simulink model "Project2"  (R2015a)
settings: Solver=ode45  StartTime=0.0  StopTime=10000  RelTol=1e-3
PreLoadFcn:
  | Init
InitFcn:
  | Init
values from neighbouring files (symbols this model uses):
  a = 5    [Init.m]
  b = 10    [Init.m]
  PACCPrecision = 32    [Init.m]
  seed = [1,2,3,4,5,6]    [Init.m]
undefined symbols (not defined in the file or in its folder): c
libraries: xbsIndex_r4 x91, xrbsComm_r4 x1
(part 1 of 2)
settings Model: Creator=chrisd  LastModifiedBy=kchilds
settings DataIOCC: SignalLoggingSaveFormat=ModelDataLogs  SignalLoggingName=sigsOut
settings OptimizationCC: BlockReduction=off  BooleanDataType=off  ExpressionDepthLimit=2147483647  InitFltsAndDblsToZero=on
settings DebuggingCC: SaveWithParameterizedLinksMsg=none  UnderspecifiedInitializationDetection=Classic  MergeDetectMultiDrivingBlocksExec=none  SignalResolutionControl=TryResolveAllWithWarning  MultiTaskDSMMsg=warning  MultiTaskCondExecSysMsg=none  FcnCallInpInsideContextMsg=UseLocalSettings  StateNameClashWarn=warning
settings HardwareCC: TargetUnknown=on
settings GRTTargetCC: TargetFcnLib=ansi_tfl_tmw.mat  ModelReferenceCompliant=off  CombineOutputUpdateFcns=off  MatFileLogging=off  GRTInterface=on

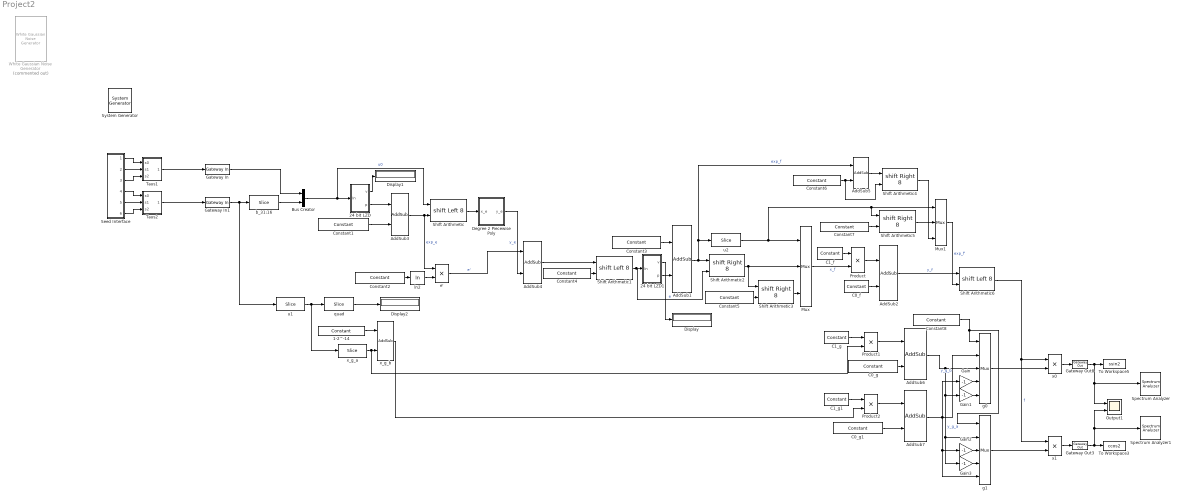
== system Project2 ==
  " System Generator" : xbsIndex_r4/ System Generator  Tag=genX  xilinxfamily=kintex7  part=xc7k325t  speed=-3  package=fbg676  synthesis_tool=Vivado  clock_wrapper=Clock Enables  directory=C:/xilinx_projects/matlab/ddc/gc4016/DDS/xilinx  proj_type=Project Navigator  Synth_file=Vivado Synthesis Defaults  Impl_file=Vivado Implementation Defaults  testbench=off  simulink_period=1  sysclk_period=7.14  dcm_input_clock_period=100  incr_netlist=off  trim_vbits=According to Block Masks  dbl_ovrd=According to Block Masks  core_generation=According to Block Masks  run_coregen=off  deprecated_control=off  eval_field=0  block_type=sysgen
      settings: block_version=12.2
  1-2^-14 : xbsIndex_r4/Constant  const=1-2^-14  gui_display_data_type=Fixed-point  arith_type=Signed (2's comp)  n_bits=LUTPrecision  bin_pt=LUTPrecisionFrc  preci_type=Single  exp_width=8  frac_width=24  explicit_period=off  period=1  equ=P=C  opselect=C  inp2=PCIN>>17  opr=+  inp1=P  carry=CIN  dbl_ovrd=off  block_type=constant
      settings: block_version=12.2
  24 bit LZD : Subsystem
  24 bit LZD1 : Subsystem
  AddSub1 : xbsIndex_r4/AddSub  mode=Subtraction  use_carryin=off  use_carryout=off  en=off  latency=0  precision=User Defined  arith_type="Signed  (2's comp)"  n_bits=nBitsIntDDSOutput  bin_pt=nBitsIntDDSOutputFrc  quantization=Truncate  overflow=Wrap  use_behavioral_HDL=off  hw_selection=Fabric  pipelined=off  dbl_ovrd=off  block_type=addsub
      settings: block_version=12.2
  AddSub{2..3,5..7} (5 alike) : xbsIndex_r4/AddSub  mode=Addition  use_carryin=off  use_carryout=off  en=off  latency=0  precision=User Defined  arith_type="Signed  (2's comp)"  n_bits=nBitsIntDDSOutput  bin_pt=nBitsIntDDSOutputFrc  quantization=Truncate  overflow=Wrap  use_behavioral_HDL=off  hw_selection=Fabric  pipelined=off  dbl_ovrd=off  block_type=addsub
      settings: block_version=12.2
  AddSub4 : xbsIndex_r4/AddSub  mode=Subtraction  use_carryin=off  use_carryout=off  en=off  latency=0  precision=User Defined  arith_type="Signed  (2's comp)"  n_bits=nBitsIntDDSOutput  bin_pt=nBitsIntDDSOutputFrc  quantization=Truncate  overflow=Wrap  use_behavioral_HDL=off  hw_selection=Fabric  pipelined=off  dbl_ovrd=off  block_type=addsub
      settings: block_version=12.2
  Bus Creator : BusCreator  Inputs=2
  C0_f : xbsIndex_r4/Constant  const=0  gui_display_data_type=Fixed-point  arith_type=Signed (2's comp)  n_bits=LUTPrecision  bin_pt=LUTPrecisionFrc  preci_type=Single  exp_width=8  frac_width=24  explicit_period=off  period=1  equ=P=C  opselect=C  inp2=PCIN>>17  opr=+  inp1=P  carry=CIN  dbl_ovrd=off  block_type=constant
      settings: block_version=12.2
  C0_g : xbsIndex_r4/Constant  const=1  gui_display_data_type=Fixed-point  arith_type=Signed (2's comp)  n_bits=LUTPrecision  bin_pt=LUTPrecisionFrc  preci_type=Single  exp_width=8  frac_width=24  explicit_period=off  period=1  equ=P=C  opselect=C  inp2=PCIN>>17  opr=+  inp1=P  carry=CIN  dbl_ovrd=off  block_type=constant
      settings: block_version=12.2
  C0_g1 : xbsIndex_r4/Constant  const=1  gui_display_data_type=Fixed-point  arith_type=Signed (2's comp)  n_bits=LUTPrecision  bin_pt=LUTPrecisionFrc  preci_type=Single  exp_width=8  frac_width=24  explicit_period=off  period=1  equ=P=C  opselect=C  inp2=PCIN>>17  opr=+  inp1=P  carry=CIN  dbl_ovrd=off  block_type=constant
      settings: block_version=12.2
  C1_f : xbsIndex_r4/Constant  const=0  gui_display_data_type=Fixed-point  arith_type=Signed (2's comp)  n_bits=LUTPrecision  bin_pt=LUTPrecisionFrc  preci_type=Single  exp_width=8  frac_width=24  explicit_period=off  period=1  equ=P=C  opselect=C  inp2=PCIN>>17  opr=+  inp1=P  carry=CIN  dbl_ovrd=off  block_type=constant
      settings: block_version=12.2
  C1_g : xbsIndex_r4/Constant  const=0  gui_display_data_type=Fixed-point  arith_type=Signed (2's comp)  n_bits=LUTPrecision  bin_pt=LUTPrecisionFrc  preci_type=Single  exp_width=8  frac_width=24  explicit_period=off  period=1  equ=P=C  opselect=C  inp2=PCIN>>17  opr=+  inp1=P  carry=CIN  dbl_ovrd=off  block_type=constant
      settings: block_version=12.2
  C1_g1 : xbsIndex_r4/Constant  const=0  gui_display_data_type=Fixed-point  arith_type=Signed (2's comp)  n_bits=LUTPrecision  bin_pt=LUTPrecisionFrc  preci_type=Single  exp_width=8  frac_width=24  explicit_period=off  period=1  equ=P=C  opselect=C  inp2=PCIN>>17  opr=+  inp1=P  carry=CIN  dbl_ovrd=off  block_type=constant
      settings: block_version=12.2
  Constant{1,4..8} (6 alike) : xbsIndex_r4/Constant  const=1  gui_display_data_type=Fixed-point  arith_type=Signed (2's comp)  n_bits=LUTPrecision  bin_pt=LUTPrecisionFrc  preci_type=Single  exp_width=8  frac_width=24  explicit_period=off  period=1  equ=P=C  opselect=C  inp2=PCIN>>17  opr=+  inp1=P  carry=CIN  dbl_ovrd=off  block_type=constant
      settings: block_version=12.2
  Constant2 : xbsIndex_r4/Constant  const=2  gui_display_data_type=Fixed-point  arith_type=Signed (2's comp)  n_bits=LUTPrecision  bin_pt=LUTPrecisionFrc  preci_type=Single  exp_width=8  frac_width=24  explicit_period=off  period=1  equ=P=C  opselect=C  inp2=PCIN>>17  opr=+  inp1=P  carry=CIN  dbl_ovrd=off  block_type=constant
      settings: block_version=12.2
  Constant3 : xbsIndex_r4/Constant  const=5  gui_display_data_type=Fixed-point  arith_type=Signed (2's comp)  n_bits=LUTPrecision  bin_pt=LUTPrecisionFrc  preci_type=Single  exp_width=8  frac_width=24  explicit_period=off  period=1  equ=P=C  opselect=C  inp2=PCIN>>17  opr=+  inp1=P  carry=CIN  dbl_ovrd=off  block_type=constant
      settings: block_version=12.2
  Degree 2 Piecewise Poly : Subsystem
  Display : Display
      settings: Format=binary (Stored Integer)
  Display1 : Display
      settings: Format=binary (Stored Integer)
  Display2 : Display
      settings: Format=binary (Stored Integer)
  Gain{,1..3} (4 alike) : Gain  Gain=-1
  Gateway In : xbsIndex_r4/Gateway In  gui_display_data_type=Fixed-point  arith_type="Signed  (2's comp)"  n_bits=32  bin_pt=0  preci_type=Single  exp_width=8  frac_width=24  rows=1  columns=1  quantization="Round  (unbiased: +/- Inf)"  overflow=Saturate  period=1  UseAsADC=off  ADCChannel='1'  interface=None  automatic_assignment=on  address_offset=hex2dec('00')  intf_name=''  intf_description=''  timing_constraint=None  locs_specified=off  LOCs={}  io_standard={}  inherit_from_input=off  hdl_port=on  dbl_ovrd=off  block_type=gatewayin
      settings: xl_area=[0, 0, 0, 0, 0, 0, 0]  block_version=VER_STRING_GOES_HERE
  Gateway In1 : xbsIndex_r4/Gateway In  gui_display_data_type=Fixed-point  arith_type="Signed  (2's comp)"  n_bits=32  bin_pt=0  preci_type=Single  exp_width=8  frac_width=24  rows=1  columns=1  quantization="Round  (unbiased: +/- Inf)"  overflow=Saturate  period=1  UseAsADC=off  ADCChannel='1'  interface=None  automatic_assignment=on  address_offset=hex2dec('00')  intf_name=''  intf_description=''  timing_constraint=None  locs_specified=off  LOCs={}  io_standard={}  inherit_from_input=off  hdl_port=on  dbl_ovrd=off  block_type=gatewayin
      settings: xl_area=[0, 0, 0, 0, 0, 0, 0]  block_version=VER_STRING_GOES_HERE
  Gateway Out3 : xbsIndex_r4/Gateway Out  inherit_from_input=off  hdl_port=on  rows=1  columns=1  UseAsDAC=off  DACChannel='1'  interface=None  automatic_assignment=on  address_offset=hex2dec('00')  intf_name=''  intf_description=''  timing_constraint=None  locs_specified=off  LOCs={}  io_standard={}  block_type=gatewayout
      settings: infoedit="Gateway out block.  Converts Xilinx fixed point inputs into ouputs of type Simulink integer, double, or fixed point.<P><P>Hardware notes:  In hardware these blocks become top level output ports or are discarded, depending on how they are configured."  xl_area=[0, 0, 0, 0, 0, 0, 0]  block_version=VER_STRING_GOES_HERE
  Gateway Out8 : xbsIndex_r4/Gateway Out  inherit_from_input=off  hdl_port=on  rows=1  columns=1  UseAsDAC=off  DACChannel='1'  interface=None  automatic_assignment=on  address_offset=hex2dec('00')  intf_name=''  intf_description=''  timing_constraint=None  locs_specified=off  LOCs={}  io_standard={}  block_type=gatewayout
      settings: infoedit="Gateway out block.  Converts Xilinx fixed point inputs into ouputs of type Simulink integer, double, or fixed point.<P><P>Hardware notes:  In hardware these blocks become top level output ports or are discarded, depending on how they are configured."  xl_area=[0, 0, 0, 0, 0, 0, 0]  block_version=VER_STRING_GOES_HERE
  Mux : xbsIndex_r4/Mux  inputs=2  en=off  latency=0  precision=Full  arith_type=Unsigned  n_bits=16  bin_pt=14  quantization=Truncate  overflow=Wrap  dbl_ovrd=off  block_type=mux
  Mux1 : xbsIndex_r4/Mux  inputs=2  en=off  latency=0  precision=Full  arith_type=Unsigned  n_bits=16  bin_pt=14  quantization=Truncate  overflow=Wrap  dbl_ovrd=off  block_type=mux
  Output1 : Scope  NumInputPorts=2
      settings: TimeRange=5000  YMin=-200000~-200000  YMax=200000~200000
  Product : Product
  Product1 : Product
  Product2 : Product
  Seed Interface : Subsystem
  Shift Arithmetic : ArithShift  BitShiftNumberSource=Input port  BitShiftNumber=8  BitShiftDirection=Left  DiagnosticForOORShift=Warning  CheckOORBitShift=on
      settings: InputPortMap=u0,p1
  Shift Arithmetic1 : ArithShift  BitShiftNumberSource=Input port  BitShiftNumber=8  BitShiftDirection=Left  DiagnosticForOORShift=Warning  CheckOORBitShift=on
      settings: InputPortMap=u0,p1
  Shift Arithmetic{2..5} (4 alike) : ArithShift  BitShiftNumberSource=Input port  BitShiftNumber=8  BitShiftDirection=Right  DiagnosticForOORShift=Warning  CheckOORBitShift=on
      settings: InputPortMap=u0,p1
  Shift Arithmetic6 : ArithShift  BitShiftNumberSource=Input port  BitShiftNumber=8  BitShiftDirection=Left  DiagnosticForOORShift=Warning  CheckOORBitShift=on
      settings: InputPortMap=u0,p1
  Spectrum Analyzer : SpectrumAnalyzer
  Spectrum Analyzer1 : SpectrumAnalyzer
  Taus1 : Subsystem
  Taus2 : Subsystem
  To Workspace3 : ToWorkspace  VariableName=ccos2  SaveFormat=Structure  SampleTime=-1
  To Workspace5 : ToWorkspace  VariableName=ssin2  SaveFormat=Structure  SampleTime=-1
  White Gaussian Noise Generator : xrbsComm_r4/White Gaussian  Noise Generator  Commented=on  seed=512
  b_31:16 : xbsIndex_r4/Slice  nbits=16  boolean_output=off  mode=Upper Bit Location + Width  bit1=0  base1=LSB of Input  bit0=PACCPrecision-1  base0=LSB of Input  dbl_ovrd=off  block_type=slice
      settings: block_version=12.2
  e' : Product
  g0 : xbsIndex_r4/Mux  inputs=4  en=off  latency=0  precision=Full  arith_type=Unsigned  n_bits=16  bin_pt=14  quantization=Truncate  overflow=Wrap  dbl_ovrd=off  block_type=mux
  g1 : xbsIndex_r4/Mux  inputs=4  en=off  latency=0  precision=Full  arith_type=Unsigned  n_bits=16  bin_pt=14  quantization=Truncate  overflow=Wrap  dbl_ovrd=off  block_type=mux
  ln2 : Math  Operator=log  OutputSignalType=real  SaturateOnIntegerOverflow=on
  quad : xbsIndex_r4/Slice  nbits=2  boolean_output=off  mode=Upper Bit Location + Width  bit1=0  base1=MSB of Input  bit0=0  base0=LSB of Input  dbl_ovrd=off  block_type=slice
      settings: block_version=12.2
  u1 : xbsIndex_r4/Slice  nbits=16  boolean_output=off  mode=Lower Bit Location + Width  bit1=0  base1=MSB of Input  bit0=0  base0=LSB of Input  dbl_ovrd=off  block_type=slice
      settings: block_version=12.2
  u2 : xbsIndex_r4/Slice  nbits=1  boolean_output=off  mode=Upper Bit Location + Width  bit1=0  base1=MSB of Input  bit0=0  base0=LSB of Input  dbl_ovrd=off  block_type=slice
      settings: block_version=12.2
  x0 : Product
  x1 : Product
  x_g_a : xbsIndex_r4/Slice  nbits=14  boolean_output=off  mode=Lower Bit Location + Width  bit1=0  base1=MSB of Input  bit0=0  base0=LSB of Input  dbl_ovrd=off  block_type=slice
      settings: block_version=12.2
  x_g_b : xbsIndex_r4/AddSub  mode=Subtraction  use_carryin=off  use_carryout=off  en=off  latency=0  precision=User Defined  arith_type="Signed  (2's comp)"  n_bits=nBitsIntDDSOutput  bin_pt=nBitsIntDDSOutputFrc  quantization=Truncate  overflow=Wrap  use_behavioral_HDL=off  hw_selection=Fabric  pipelined=off  dbl_ovrd=off  block_type=addsub
      settings: block_version=12.2
  wires:
  Gateway Out8/1 -> Spectrum Analyzer/1, Output1/1, To Workspace5/1
  Gateway In1/1 -> b_31:16/1, u1/1
  Gateway In/1 -> Bus Creator/1
  b_31:16/1 -> Bus Creator/2
  Bus Creator/1 -> Shift Arithmetic/1, 24 bit LZD/1(In)  "u0"
  Constant1/1 -> AddSub3/2
  24 bit LZD/2(p) -> AddSub3/1
  AddSub3/1 -> e'/1, Shift Arithmetic/2  "exp_e"
  Shift Arithmetic/1 -> Degree 2 Piecewise Poly/1(x_e)
  Constant2/1 -> ln2/1
  ln2/1 -> e'/2
  Degree 2 Piecewise Poly/1(y_e) -> AddSub4/2  "y_e"
  e'/1 -> AddSub4/1  "e'"
  24 bit LZD1/2(p) -> AddSub1/2
  Constant3/1 -> AddSub1/1
  AddSub4/1 -> Shift Arithmetic1/1
  Constant4/1 -> Shift Arithmetic1/2
  Shift Arithmetic1/1 -> Shift Arithmetic2/2, 24 bit LZD1/1(In)  "e"
  AddSub1/1 -> AddSub5/1, u2/1, Shift Arithmetic2/1  "exp_f"
  u2/1 -> Shift Arithmetic5/1, Mux1/1, Mux/1
  Constant5/1 -> Shift Arithmetic3/2
  Shift Arithmetic2/1 -> Mux/2, Shift Arithmetic3/1
  Shift Arithmetic3/1 -> Mux/3
  Mux/1 -> Product/2  "x_f"
  Product/1 -> AddSub2/1
  AddSub2/1 -> Shift Arithmetic6/1  "y_f"
  C0_f/1 -> AddSub2/2
  C1_f/1 -> Product/1
  Constant6/1 -> Shift Arithmetic4/2, AddSub5/2
  AddSub5/1 -> Shift Arithmetic4/1
  Shift Arithmetic4/1 -> Mux1/3
  Shift Arithmetic5/1 -> Mux1/2
  Constant7/1 -> Shift Arithmetic5/2
  Mux1/1 -> Shift Arithmetic6/2  "exp_f'"
  Shift Arithmetic6/1 -> x1/1, x0/1  "f"
  u1/1 -> x_g_a/1, quad/1
  1-2^-14/1 -> x_g_b/1
  Product1/1 -> AddSub6/1
  x_g_a/1 -> Product1/2, x_g_b/2
  C1_g/1 -> Product1/1
  C0_g/1 -> AddSub6/2
  AddSub6/1 -> Gain1/1, Gain3/1, g1/2, g0/3  "y_g_a"
  Product2/1 -> AddSub7/1
  x_g_b/1 -> Product2/2
  C1_g1/1 -> Product2/1
  C0_g1/1 -> AddSub7/2
  AddSub7/1 -> Gain/1, Gain2/1, g1/5, g0/2  "y_g_b"
  Gain/1 -> g0/4
  Gain1/1 -> g0/5
  Gain2/1 -> g1/3
  Gain3/1 -> g1/4
  g0/1 -> x0/2
  g1/1 -> x1/2
  x0/1 -> Gateway Out8/1
  x1/1 -> Gateway Out3/1
  Gateway Out3/1 -> Spectrum Analyzer1/1, Output1/2, To Workspace3/1
  24 bit LZD1/1(v) -> Display/1
  24 bit LZD/1(v) -> Display1/1
  quad/1 -> Display2/1
  Constant8/1 -> g0/1, g1/1
  Taus1/1(taus) -> Gateway In/1
  Taus2/1(taus) -> Gateway In1/1
  Seed Interface/2(Seed2) -> Taus1/2(s1)
  Seed Interface/1(Seed1) -> Taus1/1(s0)
  Seed Interface/3(Seed3) -> Taus1/3(s2)
  Seed Interface/4(Seed4) -> Taus2/1(s0)
  Seed Interface/5(Seed5) -> Taus2/2(s1)
  Seed Interface/6(Seed6) -> Taus2/3(s2)

== system Project2/24 bit LZD ==
  In : Inport
  16 bit LZD : Subsystem
  8 bit LZD : Subsystem
  Bus Creator1 : BusCreator  Inputs=2
  Demux : Demux  Outputs=24
  Logical Operator : Logic  Operator=OR  IconShape=distinctive  AllPortsSameDT=off  OutDataTypeStr=boolean
  Logical Operator2 : Logic  Operator=NOT  IconShape=distinctive  AllPortsSameDT=off  OutDataTypeStr=boolean
  Mux : Mux  Inputs=2
  v : Outport
  p : Outport  Port=2
  wires:
  Demux/8 -> 16 bit LZD/8(a7)
  Demux/10 -> 16 bit LZD/10(a9)
  In/1 -> Demux/1
  Demux/14 -> 16 bit LZD/14(a13)
  Demux/17 -> 8 bit LZD/1(a0)
  Demux/2 -> 16 bit LZD/2(a1)
  Demux/7 -> 16 bit LZD/7(a6)
  Demux/15 -> 16 bit LZD/15(a14)
  Demux/6 -> 16 bit LZD/6(a5)
  Demux/13 -> 16 bit LZD/13(a12)
  Demux/19 -> 8 bit LZD/3(a2)
  Demux/3 -> 16 bit LZD/3(a2)
  Demux/16 -> 16 bit LZD/16(a15)
  Demux/24 -> 8 bit LZD/8(a7)
  Demux/12 -> 16 bit LZD/12(a11)
  Mux/1 -> Logical Operator/2, Bus Creator1/1
  8 bit LZD/2(p) -> Mux/2
  Demux/4 -> 16 bit LZD/4(a3)
  Bus Creator1/1 -> p/1
  8 bit LZD/1(v) -> Logical Operator2/1
  Demux/1 -> 16 bit LZD/1(a0)
  Logical Operator2/1 -> Bus Creator1/2
  16 bit LZD/1(v) -> Logical Operator/1
  16 bit LZD/2(p) -> Mux/1
  Logical Operator/1 -> v/1
  Demux/9 -> 16 bit LZD/9(a8)
  Demux/5 -> 16 bit LZD/5(a4)
  Demux/11 -> 16 bit LZD/11(a10)
  Demux/23 -> 8 bit LZD/7(a6)
  Demux/20 -> 8 bit LZD/4(a3)
  Demux/22 -> 8 bit LZD/6(a5)
  Demux/21 -> 8 bit LZD/5(a4)
  Demux/18 -> 8 bit LZD/2(a1)

== system Project2/24 bit LZD1 ==
  In : Inport
  16 bit LZD : Subsystem
  8 bit LZD : Subsystem
  Bus Creator1 : BusCreator  Inputs=2
  Demux : Demux  Outputs=24
  Logical Operator : Logic  Operator=OR  IconShape=distinctive  AllPortsSameDT=off  OutDataTypeStr=boolean
  Logical Operator2 : Logic  Operator=NOT  IconShape=distinctive  AllPortsSameDT=off  OutDataTypeStr=boolean
  Mux : Mux  Inputs=2
  v : Outport
  p : Outport  Port=2
  wires:
  Demux/8 -> 16 bit LZD/8(a7)
  Demux/10 -> 16 bit LZD/10(a9)
  In/1 -> Demux/1
  Demux/14 -> 16 bit LZD/14(a13)
  Demux/17 -> 8 bit LZD/1(a0)
  Demux/2 -> 16 bit LZD/2(a1)
  Demux/7 -> 16 bit LZD/7(a6)
  Demux/15 -> 16 bit LZD/15(a14)
  Demux/6 -> 16 bit LZD/6(a5)
  Demux/13 -> 16 bit LZD/13(a12)
  Demux/19 -> 8 bit LZD/3(a2)
  Demux/3 -> 16 bit LZD/3(a2)
  Demux/16 -> 16 bit LZD/16(a15)
  Demux/24 -> 8 bit LZD/8(a7)
  Demux/12 -> 16 bit LZD/12(a11)
  Mux/1 -> Logical Operator/2, Bus Creator1/1
  8 bit LZD/2(p) -> Mux/2
  Demux/4 -> 16 bit LZD/4(a3)
  Bus Creator1/1 -> p/1
  8 bit LZD/1(v) -> Logical Operator2/1
  Demux/1 -> 16 bit LZD/1(a0)
  Logical Operator2/1 -> Bus Creator1/2
  16 bit LZD/1(v) -> Logical Operator/1
  16 bit LZD/2(p) -> Mux/1
  Logical Operator/1 -> v/1
  Demux/9 -> 16 bit LZD/9(a8)
  Demux/5 -> 16 bit LZD/5(a4)
  Demux/11 -> 16 bit LZD/11(a10)
  Demux/23 -> 8 bit LZD/7(a6)
  Demux/20 -> 8 bit LZD/4(a3)
  Demux/22 -> 8 bit LZD/6(a5)
  Demux/21 -> 8 bit LZD/5(a4)
  Demux/18 -> 8 bit LZD/2(a1)

== system Project2/Degree 2 Piecewise Poly ==
  x_e : Inport
  AddSub4 : xbsIndex_r4/AddSub  mode=Addition  use_carryin=off  use_carryout=off  en=off  latency=0  precision=User Defined  arith_type="Signed  (2's comp)"  n_bits=nBitsIntDDSOutput  bin_pt=nBitsIntDDSOutputFrc  quantization=Truncate  overflow=Wrap  use_behavioral_HDL=off  hw_selection=Fabric  pipelined=off  dbl_ovrd=off  block_type=addsub
      settings: block_version=12.2
  C1_e : xbsIndex_r4/Constant  const=0  gui_display_data_type=Fixed-point  arith_type=Signed (2's comp)  n_bits=LUTPrecision  bin_pt=LUTPrecisionFrc  preci_type=Single  exp_width=8  frac_width=24  explicit_period=off  period=1  equ=P=C  opselect=C  inp2=PCIN>>17  opr=+  inp1=P  carry=CIN  dbl_ovrd=off  block_type=constant
      settings: block_version=12.2
  C2_e : xbsIndex_r4/Constant  const=0  gui_display_data_type=Fixed-point  arith_type=Signed (2's comp)  n_bits=LUTPrecision  bin_pt=LUTPrecisionFrc  preci_type=Single  exp_width=8  frac_width=24  explicit_period=off  period=1  equ=P=C  opselect=C  inp2=PCIN>>17  opr=+  inp1=P  carry=CIN  dbl_ovrd=off  block_type=constant
      settings: block_version=12.2
  Product : Product
  Product1 : Product
  x_e_B : xbsIndex_r4/Constant  const=0  gui_display_data_type=Fixed-point  arith_type=Signed (2's comp)  n_bits=LUTPrecision  bin_pt=LUTPrecisionFrc  preci_type=Single  exp_width=8  frac_width=24  explicit_period=off  period=1  equ=P=C  opselect=C  inp2=PCIN>>17  opr=+  inp1=P  carry=CIN  dbl_ovrd=off  block_type=constant
      settings: block_version=12.2
  y_e : Outport
  wires:
  Product/1 -> AddSub4/1
  AddSub4/1 -> Product1/1
  C1_e/1 -> AddSub4/2
  x_e_B/1 -> Product1/2
  Product1/1 -> y_e/1
  x_e/1 -> Product/2
  C2_e/1 -> Product/1

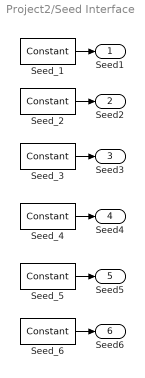
== system Project2/Seed Interface ==
  Seed_1 : xbsIndex_r4/Constant  const=seed(1)  gui_display_data_type=Fixed-point  arith_type=Signed (2's comp)  n_bits=LUTPrecision  bin_pt=LUTPrecisionFrc  preci_type=Single  exp_width=8  frac_width=24  explicit_period=off  period=1  equ=P=C  opselect=C  inp2=PCIN>>17  opr=+  inp1=P  carry=CIN  dbl_ovrd=off  block_type=constant
      settings: block_version=12.2
  Seed_2 : xbsIndex_r4/Constant  const=seed(2)  gui_display_data_type=Fixed-point  arith_type=Signed (2's comp)  n_bits=LUTPrecision  bin_pt=LUTPrecisionFrc  preci_type=Single  exp_width=8  frac_width=24  explicit_period=off  period=1  equ=P=C  opselect=C  inp2=PCIN>>17  opr=+  inp1=P  carry=CIN  dbl_ovrd=off  block_type=constant
      settings: block_version=12.2
  Seed_3 : xbsIndex_r4/Constant  const=seed(3)  gui_display_data_type=Fixed-point  arith_type=Signed (2's comp)  n_bits=LUTPrecision  bin_pt=LUTPrecisionFrc  preci_type=Single  exp_width=8  frac_width=24  explicit_period=off  period=1  equ=P=C  opselect=C  inp2=PCIN>>17  opr=+  inp1=P  carry=CIN  dbl_ovrd=off  block_type=constant
      settings: block_version=12.2
  Seed_4 : xbsIndex_r4/Constant  const=seed(4)  gui_display_data_type=Fixed-point  arith_type=Signed (2's comp)  n_bits=LUTPrecision  bin_pt=LUTPrecisionFrc  preci_type=Single  exp_width=8  frac_width=24  explicit_period=off  period=1  equ=P=C  opselect=C  inp2=PCIN>>17  opr=+  inp1=P  carry=CIN  dbl_ovrd=off  block_type=constant
      settings: block_version=12.2
  Seed_5 : xbsIndex_r4/Constant  const=seed(5)  gui_display_data_type=Fixed-point  arith_type=Signed (2's comp)  n_bits=LUTPrecision  bin_pt=LUTPrecisionFrc  preci_type=Single  exp_width=8  frac_width=24  explicit_period=off  period=1  equ=P=C  opselect=C  inp2=PCIN>>17  opr=+  inp1=P  carry=CIN  dbl_ovrd=off  block_type=constant
      settings: block_version=12.2
  Seed_6 : xbsIndex_r4/Constant  const=seed(6)  gui_display_data_type=Fixed-point  arith_type=Signed (2's comp)  n_bits=LUTPrecision  bin_pt=LUTPrecisionFrc  preci_type=Single  exp_width=8  frac_width=24  explicit_period=off  period=1  equ=P=C  opselect=C  inp2=PCIN>>17  opr=+  inp1=P  carry=CIN  dbl_ovrd=off  block_type=constant
      settings: block_version=12.2
  Seed1 : Outport
  Seed2 : Outport  Port=2
  Seed3 : Outport  Port=3
  Seed4 : Outport  Port=4
  Seed5 : Outport  Port=5
  Seed6 : Outport  Port=6
  wires:
  Seed_4/1 -> Seed4/1
  Seed_1/1 -> Seed1/1
  Seed_2/1 -> Seed2/1
  Seed_3/1 -> Seed3/1
  Seed_6/1 -> Seed6/1
  Seed_5/1 -> Seed5/1

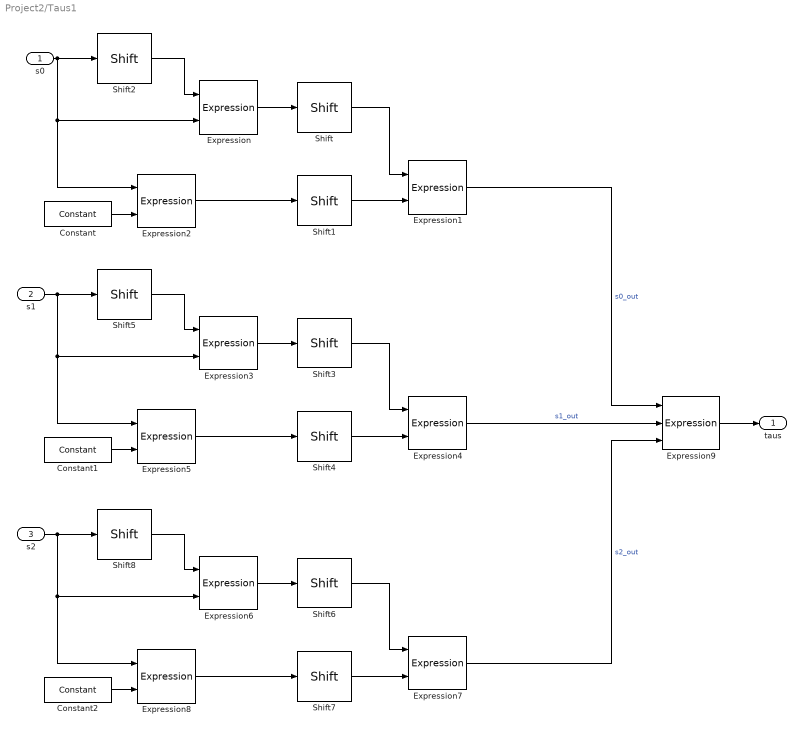
== system Project2/Taus1 ==
  s0 : Inport
  s1 : Inport  Port=2
  s2 : Inport  Port=3
  Constant : xbsIndex_r4/Constant  const=hex2dec('fffffffe')  gui_display_data_type=Floating-point  arith_type=Floating-point  n_bits=16  bin_pt=14  preci_type=Double  exp_width=8  frac_width=24  explicit_period=off  period=1  equ=P=C  opselect=C  inp2=PCIN>>17  opr=+  inp1=P  carry=CIN  dbl_ovrd=off  block_type=constant
  Constant1 : xbsIndex_r4/Constant  const=hex2dec('fffffff8')  gui_display_data_type=Floating-point  arith_type=Floating-point  n_bits=16  bin_pt=14  preci_type=Double  exp_width=8  frac_width=24  explicit_period=off  period=1  equ=P=C  opselect=C  inp2=PCIN>>17  opr=+  inp1=P  carry=CIN  dbl_ovrd=off  block_type=constant
  Constant2 : xbsIndex_r4/Constant  const=hex2dec('fffffff0')  gui_display_data_type=Floating-point  arith_type=Floating-point  n_bits=16  bin_pt=14  preci_type=Double  exp_width=8  frac_width=24  explicit_period=off  period=1  equ=P=C  opselect=C  inp2=PCIN>>17  opr=+  inp1=P  carry=CIN  dbl_ovrd=off  block_type=constant
  Expression{,1,3..4,6..7} (6 alike) : xbsIndex_r4/Expression  expression=a ^ b  align_bp=on  en=off  latency=0  precision=Full  arith_type=Unsigned  n_bits=16  bin_pt=0  dbl_ovrd=off  block_type=expr
  Expression2 : xbsIndex_r4/Expression  expression=a & b  align_bp=on  en=off  latency=0  precision=Full  arith_type=Unsigned  n_bits=16  bin_pt=0  dbl_ovrd=off  block_type=expr
  Expression5 : xbsIndex_r4/Expression  expression=a & b  align_bp=on  en=off  latency=0  precision=Full  arith_type=Unsigned  n_bits=16  bin_pt=0  dbl_ovrd=off  block_type=expr
  Expression8 : xbsIndex_r4/Expression  expression=a & b  align_bp=on  en=off  latency=0  precision=Full  arith_type=Unsigned  n_bits=16  bin_pt=0  dbl_ovrd=off  block_type=expr
  Expression9 : xbsIndex_r4/Expression  expression=a ^ b ^ c  align_bp=on  en=off  latency=0  precision=Full  arith_type=Unsigned  n_bits=16  bin_pt=0  dbl_ovrd=off  block_type=expr
  Shift : xbsIndex_r4/Shift  shift_dir=Right  shift_bits=19  en=off  latency=0  precision=Full  arith_type="Signed  (2's comp)"  n_bits=16  bin_pt=14  quantization=Truncate  overflow=Wrap  dbl_ovrd=off  block_type=shift
  Shift1 : xbsIndex_r4/Shift  shift_dir=Left  shift_bits=12  en=off  latency=0  precision=Full  arith_type="Signed  (2's comp)"  n_bits=16  bin_pt=14  quantization=Truncate  overflow=Wrap  dbl_ovrd=off  block_type=shift
  Shift2 : xbsIndex_r4/Shift  shift_dir=Left  shift_bits=13  en=off  latency=0  precision=Full  arith_type="Signed  (2's comp)"  n_bits=16  bin_pt=14  quantization=Truncate  overflow=Wrap  dbl_ovrd=off  block_type=shift
  Shift3 : xbsIndex_r4/Shift  shift_dir=Right  shift_bits=25  en=off  latency=0  precision=Full  arith_type="Signed  (2's comp)"  n_bits=16  bin_pt=14  quantization=Truncate  overflow=Wrap  dbl_ovrd=off  block_type=shift
  Shift4 : xbsIndex_r4/Shift  shift_dir=Left  shift_bits=4  en=off  latency=0  precision=Full  arith_type="Signed  (2's comp)"  n_bits=16  bin_pt=14  quantization=Truncate  overflow=Wrap  dbl_ovrd=off  block_type=shift
  Shift5 : xbsIndex_r4/Shift  shift_dir=Left  shift_bits=2  en=off  latency=0  precision=Full  arith_type="Signed  (2's comp)"  n_bits=16  bin_pt=14  quantization=Truncate  overflow=Wrap  dbl_ovrd=off  block_type=shift
  Shift6 : xbsIndex_r4/Shift  shift_dir=Right  shift_bits=11  en=off  latency=0  precision=Full  arith_type="Signed  (2's comp)"  n_bits=16  bin_pt=14  quantization=Truncate  overflow=Wrap  dbl_ovrd=off  block_type=shift
  Shift7 : xbsIndex_r4/Shift  shift_dir=Left  shift_bits=17  en=off  latency=0  precision=Full  arith_type="Signed  (2's comp)"  n_bits=16  bin_pt=14  quantization=Truncate  overflow=Wrap  dbl_ovrd=off  block_type=shift
  Shift8 : xbsIndex_r4/Shift  shift_dir=Left  shift_bits=3  en=off  latency=0  precision=Full  arith_type="Signed  (2's comp)"  n_bits=16  bin_pt=14  quantization=Truncate  overflow=Wrap  dbl_ovrd=off  block_type=shift
  taus : Outport
  wires:
  Shift2/1 -> Expression/1
  s0/1 -> Shift2/1, Expression2/1, Expression/2
  Expression/1 -> Shift/1
  Shift/1 -> Expression1/1
  Expression2/1 -> Shift1/1
  Shift1/1 -> Expression1/2
  Constant/1 -> Expression2/2
  Expression1/1 -> Expression9/1  "s0_out"
  Shift5/1 -> Expression3/1
  s1/1 -> Expression3/2, Expression5/1, Shift5/1
  Expression3/1 -> Shift3/1
  Shift3/1 -> Expression4/1
  Expression5/1 -> Shift4/1
  Shift4/1 -> Expression4/2
  Constant1/1 -> Expression5/2
  Expression4/1 -> Expression9/2  "s1_out"
  Shift8/1 -> Expression6/1
  s2/1 -> Expression6/2, Expression8/1, Shift8/1
  Expression6/1 -> Shift6/1
  Shift6/1 -> Expression7/1
  Expression8/1 -> Shift7/1
  Shift7/1 -> Expression7/2
  Constant2/1 -> Expression8/2
  Expression7/1 -> Expression9/3  "s2_out"
  Expression9/1 -> taus/1

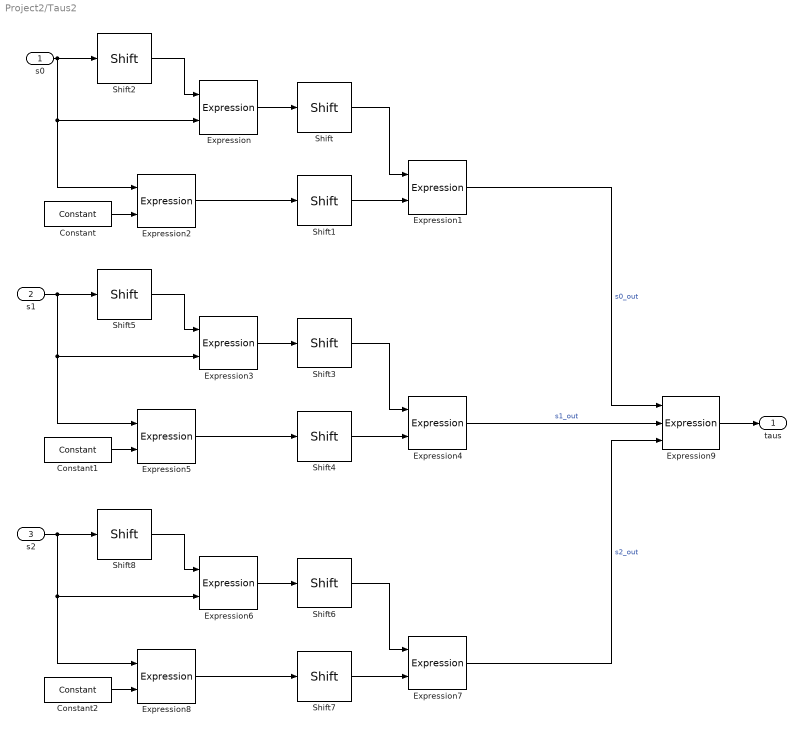
== system Project2/Taus2 ==
  s0 : Inport
  s1 : Inport  Port=2
  s2 : Inport  Port=3
  Constant : xbsIndex_r4/Constant  const=hex2dec('fffffffe')  gui_display_data_type=Floating-point  arith_type=Floating-point  n_bits=16  bin_pt=14  preci_type=Double  exp_width=8  frac_width=24  explicit_period=off  period=1  equ=P=C  opselect=C  inp2=PCIN>>17  opr=+  inp1=P  carry=CIN  dbl_ovrd=off  block_type=constant
  Constant1 : xbsIndex_r4/Constant  const=hex2dec('fffffff8')  gui_display_data_type=Floating-point  arith_type=Floating-point  n_bits=16  bin_pt=14  preci_type=Double  exp_width=8  frac_width=24  explicit_period=off  period=1  equ=P=C  opselect=C  inp2=PCIN>>17  opr=+  inp1=P  carry=CIN  dbl_ovrd=off  block_type=constant
  Constant2 : xbsIndex_r4/Constant  const=hex2dec('fffffff0')  gui_display_data_type=Floating-point  arith_type=Floating-point  n_bits=16  bin_pt=14  preci_type=Double  exp_width=8  frac_width=24  explicit_period=off  period=1  equ=P=C  opselect=C  inp2=PCIN>>17  opr=+  inp1=P  carry=CIN  dbl_ovrd=off  block_type=constant
  Expression{,1,3..4,6..7} (6 alike) : xbsIndex_r4/Expression  expression=a ^ b  align_bp=on  en=off  latency=0  precision=Full  arith_type=Unsigned  n_bits=16  bin_pt=0  dbl_ovrd=off  block_type=expr
  Expression2 : xbsIndex_r4/Expression  expression=a & b  align_bp=on  en=off  latency=0  precision=Full  arith_type=Unsigned  n_bits=16  bin_pt=0  dbl_ovrd=off  block_type=expr
  Expression5 : xbsIndex_r4/Expression  expression=a & b  align_bp=on  en=off  latency=0  precision=Full  arith_type=Unsigned  n_bits=16  bin_pt=0  dbl_ovrd=off  block_type=expr
  Expression8 : xbsIndex_r4/Expression  expression=a & b  align_bp=on  en=off  latency=0  precision=Full  arith_type=Unsigned  n_bits=16  bin_pt=0  dbl_ovrd=off  block_type=expr
  Expression9 : xbsIndex_r4/Expression  expression=a ^ b ^ c  align_bp=on  en=off  latency=0  precision=Full  arith_type=Unsigned  n_bits=16  bin_pt=0  dbl_ovrd=off  block_type=expr
  Shift : xbsIndex_r4/Shift  shift_dir=Right  shift_bits=19  en=off  latency=0  precision=Full  arith_type="Signed  (2's comp)"  n_bits=16  bin_pt=14  quantization=Truncate  overflow=Wrap  dbl_ovrd=off  block_type=shift
  Shift1 : xbsIndex_r4/Shift  shift_dir=Left  shift_bits=12  en=off  latency=0  precision=Full  arith_type="Signed  (2's comp)"  n_bits=16  bin_pt=14  quantization=Truncate  overflow=Wrap  dbl_ovrd=off  block_type=shift
  Shift2 : xbsIndex_r4/Shift  shift_dir=Left  shift_bits=13  en=off  latency=0  precision=Full  arith_type="Signed  (2's comp)"  n_bits=16  bin_pt=14  quantization=Truncate  overflow=Wrap  dbl_ovrd=off  block_type=shift
  Shift3 : xbsIndex_r4/Shift  shift_dir=Right  shift_bits=25  en=off  latency=0  precision=Full  arith_type="Signed  (2's comp)"  n_bits=16  bin_pt=14  quantization=Truncate  overflow=Wrap  dbl_ovrd=off  block_type=shift
  Shift4 : xbsIndex_r4/Shift  shift_dir=Left  shift_bits=4  en=off  latency=0  precision=Full  arith_type="Signed  (2's comp)"  n_bits=16  bin_pt=14  quantization=Truncate  overflow=Wrap  dbl_ovrd=off  block_type=shift
  Shift5 : xbsIndex_r4/Shift  shift_dir=Left  shift_bits=2  en=off  latency=0  precision=Full  arith_type="Signed  (2's comp)"  n_bits=16  bin_pt=14  quantization=Truncate  overflow=Wrap  dbl_ovrd=off  block_type=shift
  Shift6 : xbsIndex_r4/Shift  shift_dir=Right  shift_bits=11  en=off  latency=0  precision=Full  arith_type="Signed  (2's comp)"  n_bits=16  bin_pt=14  quantization=Truncate  overflow=Wrap  dbl_ovrd=off  block_type=shift
  Shift7 : xbsIndex_r4/Shift  shift_dir=Left  shift_bits=17  en=off  latency=0  precision=Full  arith_type="Signed  (2's comp)"  n_bits=16  bin_pt=14  quantization=Truncate  overflow=Wrap  dbl_ovrd=off  block_type=shift
  Shift8 : xbsIndex_r4/Shift  shift_dir=Left  shift_bits=3  en=off  latency=0  precision=Full  arith_type="Signed  (2's comp)"  n_bits=16  bin_pt=14  quantization=Truncate  overflow=Wrap  dbl_ovrd=off  block_type=shift
  taus : Outport
  wires:
  Shift2/1 -> Expression/1
  s0/1 -> Shift2/1, Expression2/1, Expression/2
  Expression/1 -> Shift/1
  Shift/1 -> Expression1/1
  Expression2/1 -> Shift1/1
  Shift1/1 -> Expression1/2
  Constant/1 -> Expression2/2
  Expression1/1 -> Expression9/1  "s0_out"
  Shift5/1 -> Expression3/1
  s1/1 -> Expression3/2, Expression5/1, Shift5/1
  Expression3/1 -> Shift3/1
  Shift3/1 -> Expression4/1
  Expression5/1 -> Shift4/1
  Shift4/1 -> Expression4/2
  Constant1/1 -> Expression5/2
  Expression4/1 -> Expression9/2  "s1_out"
  Shift8/1 -> Expression6/1
  s2/1 -> Expression6/2, Expression8/1, Shift8/1
  Expression6/1 -> Shift6/1
  Shift6/1 -> Expression7/1
  Expression8/1 -> Shift7/1
  Shift7/1 -> Expression7/2
  Constant2/1 -> Expression8/2
  Expression7/1 -> Expression9/3  "s2_out"
  Expression9/1 -> taus/1

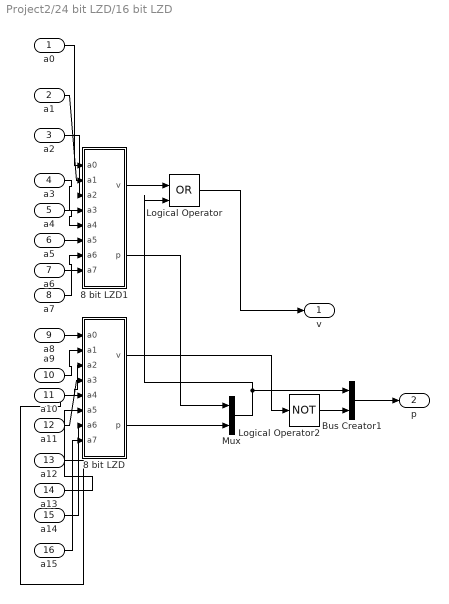
== system Project2/24 bit LZD/16 bit LZD ==
  a0 : Inport
  a1 : Inport  Port=2
  a2 : Inport  Port=3
  a3 : Inport  Port=4
  a4 : Inport  Port=5
  a5 : Inport  Port=6
  a6 : Inport  Port=7
  a7 : Inport  Port=8
  a8 : Inport  Port=9
  a9 : Inport  Port=10
  a10 : Inport  Port=11
  a11 : Inport  Port=12
  a12 : Inport  Port=13
  a13 : Inport  Port=14
  a14 : Inport  Port=15
  a15 : Inport  Port=16
  8 bit LZD : Subsystem
  8 bit LZD1 : Subsystem
  Bus Creator1 : BusCreator  Inputs=2
  Logical Operator : Logic  Operator=OR  IconShape=distinctive  AllPortsSameDT=off  OutDataTypeStr=boolean
  Logical Operator2 : Logic  Operator=NOT  IconShape=distinctive  AllPortsSameDT=off  OutDataTypeStr=boolean
  Mux : Mux  Inputs=2
  v : Outport
  p : Outport  Port=2
  wires:
  8 bit LZD/2(p) -> Mux/2
  Mux/1 -> Logical Operator/2, Bus Creator1/1
  Logical Operator2/1 -> Bus Creator1/2
  8 bit LZD/1(v) -> Logical Operator2/1
  Logical Operator/1 -> v/1
  8 bit LZD1/2(p) -> Mux/1
  Bus Creator1/1 -> p/1
  8 bit LZD1/1(v) -> Logical Operator/1
  a9/1 -> 8 bit LZD/2(a1)
  a0/1 -> 8 bit LZD1/1(a0)
  a4/1 -> 8 bit LZD1/5(a4)
  a2/1 -> 8 bit LZD1/3(a2)
  a5/1 -> 8 bit LZD1/6(a5)
  a10/1 -> 8 bit LZD/3(a2)
  a11/1 -> 8 bit LZD/4(a3)
  a8/1 -> 8 bit LZD/1(a0)
  a3/1 -> 8 bit LZD1/4(a3)
  a12/1 -> 8 bit LZD/5(a4)
  a6/1 -> 8 bit LZD1/7(a6)
  a7/1 -> 8 bit LZD1/8(a7)
  a1/1 -> 8 bit LZD1/2(a1)
  a15/1 -> 8 bit LZD/8(a7)
  a13/1 -> 8 bit LZD/6(a5)
  a14/1 -> 8 bit LZD/7(a6)

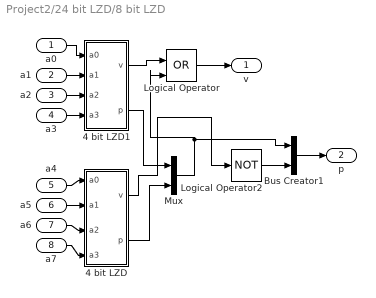
== system Project2/24 bit LZD/8 bit LZD ==
  a0 : Inport
  a1 : Inport  Port=2
  a2 : Inport  Port=3
  a3 : Inport  Port=4
  a4 : Inport  Port=5
  a5 : Inport  Port=6
  a6 : Inport  Port=7
  a7 : Inport  Port=8
  4 bit LZD : Subsystem
  4 bit LZD1 : Subsystem
  Bus Creator1 : BusCreator  Inputs=2
  Logical Operator : Logic  Operator=OR  IconShape=distinctive  AllPortsSameDT=off  OutDataTypeStr=boolean
  Logical Operator2 : Logic  Operator=NOT  IconShape=distinctive  AllPortsSameDT=off  OutDataTypeStr=boolean
  Mux : Mux  Inputs=2
  v : Outport
  p : Outport  Port=2
  wires:
  a2/1 -> 4 bit LZD1/3(a2)
  a6/1 -> 4 bit LZD/3(a2)
  a7/1 -> 4 bit LZD/4(a3)
  a3/1 -> 4 bit LZD1/4(a3)
  a0/1 -> 4 bit LZD1/1(a0)
  a1/1 -> 4 bit LZD1/2(a1)
  a5/1 -> 4 bit LZD/2(a1)
  a4/1 -> 4 bit LZD/1(a0)
  Logical Operator/1 -> v/1
  Logical Operator2/1 -> Bus Creator1/2
  4 bit LZD1/1(v) -> Logical Operator/1
  Mux/1 -> Logical Operator/2, Bus Creator1/1
  4 bit LZD/2(p) -> Mux/2
  Bus Creator1/1 -> p/1
  4 bit LZD/1(v) -> Logical Operator2/1
  4 bit LZD1/2(p) -> Mux/1

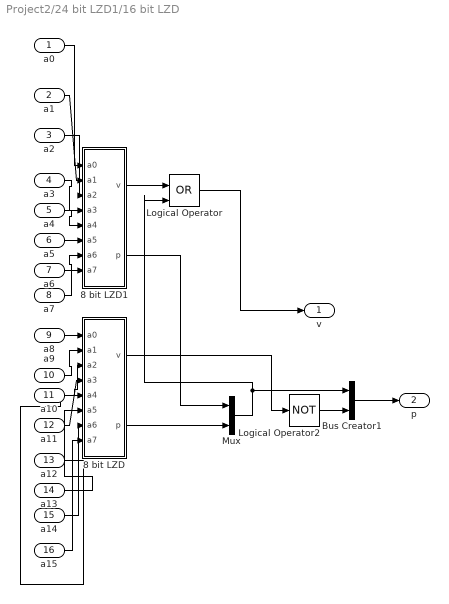
== system Project2/24 bit LZD1/16 bit LZD ==
  a0 : Inport
  a1 : Inport  Port=2
  a2 : Inport  Port=3
  a3 : Inport  Port=4
  a4 : Inport  Port=5
  a5 : Inport  Port=6
  a6 : Inport  Port=7
  a7 : Inport  Port=8
  a8 : Inport  Port=9
  a9 : Inport  Port=10
  a10 : Inport  Port=11
  a11 : Inport  Port=12
  a12 : Inport  Port=13
  a13 : Inport  Port=14
  a14 : Inport  Port=15
  a15 : Inport  Port=16
  8 bit LZD : Subsystem
  8 bit LZD1 : Subsystem
  Bus Creator1 : BusCreator  Inputs=2
  Logical Operator : Logic  Operator=OR  IconShape=distinctive  AllPortsSameDT=off  OutDataTypeStr=boolean
  Logical Operator2 : Logic  Operator=NOT  IconShape=distinctive  AllPortsSameDT=off  OutDataTypeStr=boolean
  Mux : Mux  Inputs=2
  v : Outport
  p : Outport  Port=2
  wires:
  8 bit LZD/2(p) -> Mux/2
  Mux/1 -> Logical Operator/2, Bus Creator1/1
  Logical Operator2/1 -> Bus Creator1/2
  8 bit LZD/1(v) -> Logical Operator2/1
  Logical Operator/1 -> v/1
  8 bit LZD1/2(p) -> Mux/1
  Bus Creator1/1 -> p/1
  8 bit LZD1/1(v) -> Logical Operator/1
  a9/1 -> 8 bit LZD/2(a1)
  a0/1 -> 8 bit LZD1/1(a0)
  a4/1 -> 8 bit LZD1/5(a4)
  a2/1 -> 8 bit LZD1/3(a2)
  a5/1 -> 8 bit LZD1/6(a5)
  a10/1 -> 8 bit LZD/3(a2)
  a11/1 -> 8 bit LZD/4(a3)
  a8/1 -> 8 bit LZD/1(a0)
  a3/1 -> 8 bit LZD1/4(a3)
  a12/1 -> 8 bit LZD/5(a4)
  a6/1 -> 8 bit LZD1/7(a6)
  a7/1 -> 8 bit LZD1/8(a7)
  a1/1 -> 8 bit LZD1/2(a1)
  a15/1 -> 8 bit LZD/8(a7)
  a13/1 -> 8 bit LZD/6(a5)
  a14/1 -> 8 bit LZD/7(a6)

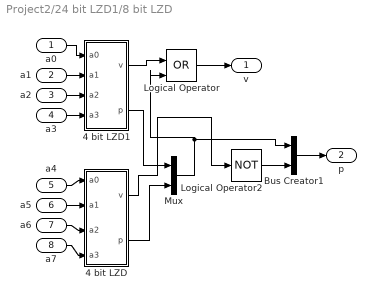
== system Project2/24 bit LZD1/8 bit LZD ==
  a0 : Inport
  a1 : Inport  Port=2
  a2 : Inport  Port=3
  a3 : Inport  Port=4
  a4 : Inport  Port=5
  a5 : Inport  Port=6
  a6 : Inport  Port=7
  a7 : Inport  Port=8
  4 bit LZD : Subsystem
  4 bit LZD1 : Subsystem
  Bus Creator1 : BusCreator  Inputs=2
  Logical Operator : Logic  Operator=OR  IconShape=distinctive  AllPortsSameDT=off  OutDataTypeStr=boolean
  Logical Operator2 : Logic  Operator=NOT  IconShape=distinctive  AllPortsSameDT=off  OutDataTypeStr=boolean
  Mux : Mux  Inputs=2
  v : Outport
  p : Outport  Port=2
  wires:
  a2/1 -> 4 bit LZD1/3(a2)
  a6/1 -> 4 bit LZD/3(a2)
  a7/1 -> 4 bit LZD/4(a3)
  a3/1 -> 4 bit LZD1/4(a3)
  a0/1 -> 4 bit LZD1/1(a0)
  a1/1 -> 4 bit LZD1/2(a1)
  a5/1 -> 4 bit LZD/2(a1)
  a4/1 -> 4 bit LZD/1(a0)
  Logical Operator/1 -> v/1
  Logical Operator2/1 -> Bus Creator1/2
  4 bit LZD1/1(v) -> Logical Operator/1
  Mux/1 -> Logical Operator/2, Bus Creator1/1
  4 bit LZD/2(p) -> Mux/2
  Bus Creator1/1 -> p/1
  4 bit LZD/1(v) -> Logical Operator2/1
  4 bit LZD1/2(p) -> Mux/1

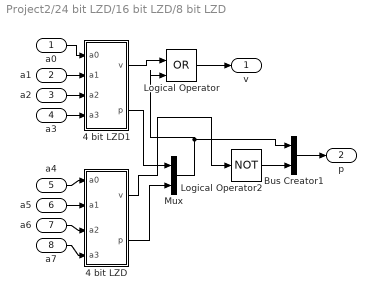
== system Project2/24 bit LZD/16 bit LZD/8 bit LZD ==
  a0 : Inport
  a1 : Inport  Port=2
  a2 : Inport  Port=3
  a3 : Inport  Port=4
  a4 : Inport  Port=5
  a5 : Inport  Port=6
  a6 : Inport  Port=7
  a7 : Inport  Port=8
  4 bit LZD : Subsystem
  4 bit LZD1 : Subsystem
  Bus Creator1 : BusCreator  Inputs=2
  Logical Operator : Logic  Operator=OR  IconShape=distinctive  AllPortsSameDT=off  OutDataTypeStr=boolean
  Logical Operator2 : Logic  Operator=NOT  IconShape=distinctive  AllPortsSameDT=off  OutDataTypeStr=boolean
  Mux : Mux  Inputs=2
  v : Outport
  p : Outport  Port=2
  wires:
  a2/1 -> 4 bit LZD1/3(a2)
  a6/1 -> 4 bit LZD/3(a2)
  a7/1 -> 4 bit LZD/4(a3)
  a3/1 -> 4 bit LZD1/4(a3)
  a0/1 -> 4 bit LZD1/1(a0)
  a1/1 -> 4 bit LZD1/2(a1)
  a5/1 -> 4 bit LZD/2(a1)
  a4/1 -> 4 bit LZD/1(a0)
  Logical Operator/1 -> v/1
  Logical Operator2/1 -> Bus Creator1/2
  4 bit LZD1/1(v) -> Logical Operator/1
  Mux/1 -> Logical Operator/2, Bus Creator1/1
  4 bit LZD/2(p) -> Mux/2
  Bus Creator1/1 -> p/1
  4 bit LZD/1(v) -> Logical Operator2/1
  4 bit LZD1/2(p) -> Mux/1

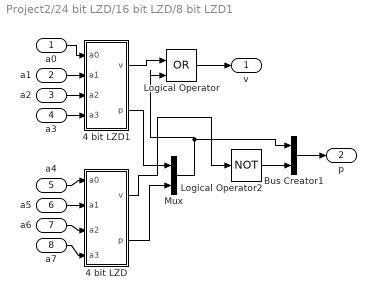
== system Project2/24 bit LZD/16 bit LZD/8 bit LZD1 ==
  a0 : Inport
  a1 : Inport  Port=2
  a2 : Inport  Port=3
  a3 : Inport  Port=4
  a4 : Inport  Port=5
  a5 : Inport  Port=6
  a6 : Inport  Port=7
  a7 : Inport  Port=8
  4 bit LZD : Subsystem
  4 bit LZD1 : Subsystem
  Bus Creator1 : BusCreator  Inputs=2
  Logical Operator : Logic  Operator=OR  IconShape=distinctive  AllPortsSameDT=off  OutDataTypeStr=boolean
  Logical Operator2 : Logic  Operator=NOT  IconShape=distinctive  AllPortsSameDT=off  OutDataTypeStr=boolean
  Mux : Mux  Inputs=2
  v : Outport
  p : Outport  Port=2
  wires:
  a2/1 -> 4 bit LZD1/3(a2)
  a6/1 -> 4 bit LZD/3(a2)
  a7/1 -> 4 bit LZD/4(a3)
  a3/1 -> 4 bit LZD1/4(a3)
  a0/1 -> 4 bit LZD1/1(a0)
  a1/1 -> 4 bit LZD1/2(a1)
  a5/1 -> 4 bit LZD/2(a1)
  a4/1 -> 4 bit LZD/1(a0)
  Logical Operator/1 -> v/1
  Logical Operator2/1 -> Bus Creator1/2
  4 bit LZD1/1(v) -> Logical Operator/1
  Mux/1 -> Logical Operator/2, Bus Creator1/1
  4 bit LZD/2(p) -> Mux/2
  Bus Creator1/1 -> p/1
  4 bit LZD/1(v) -> Logical Operator2/1
  4 bit LZD1/2(p) -> Mux/1

== system Project2/24 bit LZD/8 bit LZD/4 bit LZD ==
  a0 : Inport
  a1 : Inport  Port=2
  a2 : Inport  Port=3
  a3 : Inport  Port=4
  2 bit LZD : Subsystem
  2 bit LZD1 : Subsystem
  Bus Creator1 : BusCreator  Inputs=2
  Logical Operator : Logic  Operator=OR  IconShape=distinctive  AllPortsSameDT=off  OutDataTypeStr=boolean
  Logical Operator2 : Logic  Operator=NOT  IconShape=distinctive  AllPortsSameDT=off  OutDataTypeStr=boolean
  Mux : Mux  Inputs=2
  v : Outport
  p : Outport  Port=2
  wires:
  2 bit LZD/1(v) -> Logical Operator2/1
  2 bit LZD1/2(p) -> Mux/1
  2 bit LZD/2(p) -> Mux/2
  Bus Creator1/1 -> p/1
  a0/1 -> 2 bit LZD1/1(a0)
  a2/1 -> 2 bit LZD/1(a0)
  a1/1 -> 2 bit LZD1/2(a1)
  a3/1 -> 2 bit LZD/2(a1)
  Logical Operator/1 -> v/1
  2 bit LZD1/1(v) -> Logical Operator/1
  Logical Operator2/1 -> Bus Creator1/2
  Mux/1 -> Logical Operator/2, Bus Creator1/1

== system Project2/24 bit LZD/8 bit LZD/4 bit LZD1 ==
  a0 : Inport
  a1 : Inport  Port=2
  a2 : Inport  Port=3
  a3 : Inport  Port=4
  2 bit LZD : Subsystem
  2 bit LZD1 : Subsystem
  Bus Creator1 : BusCreator  Inputs=2
  Logical Operator : Logic  Operator=OR  IconShape=distinctive  AllPortsSameDT=off  OutDataTypeStr=boolean
  Logical Operator2 : Logic  Operator=NOT  IconShape=distinctive  AllPortsSameDT=off  OutDataTypeStr=boolean
  Mux : Mux  Inputs=2
  v : Outport
  p : Outport  Port=2
  wires:
  2 bit LZD/1(v) -> Logical Operator2/1
  2 bit LZD1/2(p) -> Mux/1
  2 bit LZD/2(p) -> Mux/2
  Bus Creator1/1 -> p/1
  a0/1 -> 2 bit LZD1/1(a0)
  a2/1 -> 2 bit LZD/1(a0)
  a1/1 -> 2 bit LZD1/2(a1)
  a3/1 -> 2 bit LZD/2(a1)
  Logical Operator/1 -> v/1
  2 bit LZD1/1(v) -> Logical Operator/1
  Logical Operator2/1 -> Bus Creator1/2
  Mux/1 -> Logical Operator/2, Bus Creator1/1
